simulink model "gm_sampleModel1569_sub"  (R2023a)
settings: Solver=VariableStepAuto  StartTime=0.0  StopTime=10.0  RelTol=1e-3
libraries: hdlsllib x2, simulink x1
settings Model: Creator=user1  LastModifiedBy=user1
settings OptimizationCC: BlockReduction=off  ConditionallyExecuteInputs=off
settings DebuggingCC: InheritedTsInSrcMsg=none

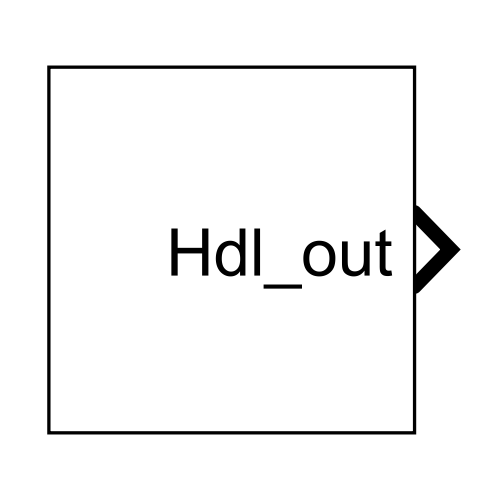
[thumbnail: Simulink's stored preview of the top-level diagram]
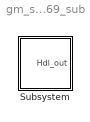
== system gm_sampleModel1569_sub ==
  Subsystem : Subsystem

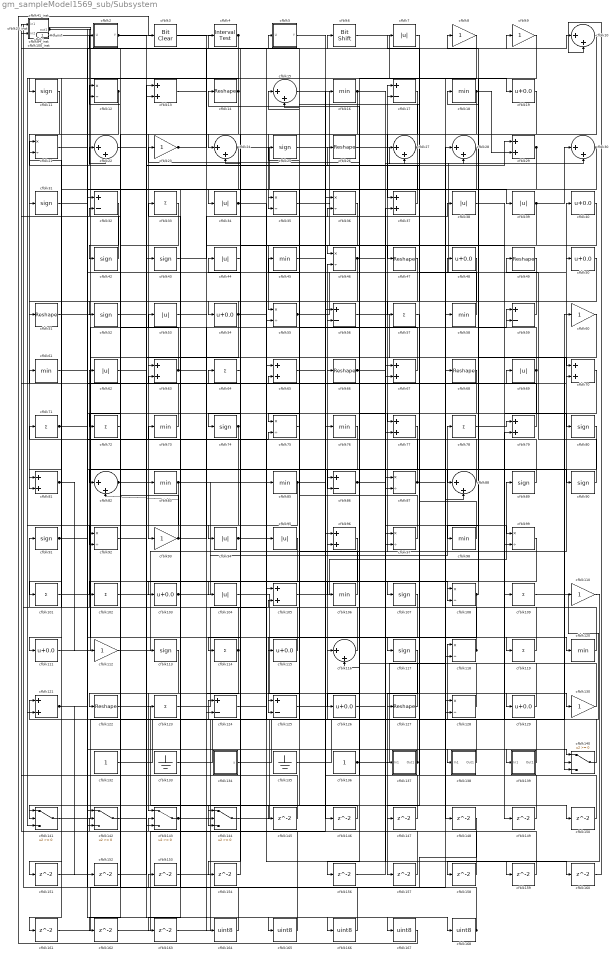
== system gm_sampleModel1569_sub/Subsystem ==
  cfblk1 : Constant  Value=0  OutDataTypeStr=uint8  SampleTime=1
  cfblk{10,15,22,24,27..28,30,82,88,116} (10 alike) : Sum  Inputs=|++  OutDataTypeStr=uint8
  cfblk100_inst : Subsystem
  cfblk{33,57,64,71..72,78,101..102,109,114,119,123} (12 alike) : Sum  Inputs=+  OutDataTypeStr=uint8
  cfblk{19,40,48,50,54,103,111,115,126,129} (10 alike) : Bias  Bias=0.0  SaturateOnIntegerOverflow=off
  cfblk{7,34,38..39,44,53,62,69,94..95,104} (11 alike) : Abs  OutDataTypeStr=uint8  SaturateOnIntegerOverflow=off
  cfblk{13,29,37,63,65,67,70,77,79,81,96,105,121} (13 alike) : Sum  OutDataTypeStr=uint8
  cfblk{16,18,45,58,61,73,76,83,85,98,106,120} (12 alike) : MinMax  OutDataTypeStr=uint8
  cfblk{11,25,31,42..43,52,74,80,89..91,107,113,117} (14 alike) : Signum
  cfblk{12,21,35..36,46,55,75,87,92,97,99,108,118,128} (14 alike) : Product  Inputs=*/  OutDataTypeStr=uint8  RndMeth=Zero  SaturateOnIntegerOverflow=on
  cfblk{8..9,23,60,93,110,112,130} (8 alike) : Gain  OutDataTypeStr=uint8
  cfblk{14,26,47,49,51,66,68,122,127} (9 alike) : Reshape
  cfblk{17,32,56,59,86,124..125} (7 alike) : Sum  Inputs=+-  OutDataTypeStr=uint8
  cfblk132 : Constant  OutDataTypeStr=uint8  SampleTime=-1
  cfblk133 : Ground
  cfblk134 : Subsystem  mask(Counter Free-Running){NumBits=double(16), tsamp=double(-1)}
      mask prompts: NumBits "Simulink:masks:NumberOfBits_MP"; tsamp "Simulink:masks:SampleTime_MP"
      mask help: Simulink:masks:CounterFreeRunning_MD
  cfblk135 : Ground
  cfblk136 : Constant  OutDataTypeStr=uint8  SampleTime=-1
  cfblk137 : Subsystem
  cfblk138 : Subsystem
  cfblk139 : Subsystem
  cfblk{140..144} (5 alike) : Switch  OutDataTypeStr=uint8  SaturateOnIntegerOverflow=off  InputSameDT=off
  cfblk{145..154,156..163} (18 alike) : Delay  SampleTime=1
  cfblk{164..168} (5 alike) : DataTypeConversion  OutDataTypeStr=uint8  SaturateOnIntegerOverflow=off  RndMeth=Floor
  cfblk2 : Subsystem  mask(Detect Fall Negative){vinit=double(0), InputProcessing=Elements as channels (sample based), OutDataTypeStr=uint8}
      mask prompts: vinit "Simulink:masks:InitialCondition_MP"; InputProcessing "Simulink:masks:InputProcessing_MP"; OutDataTypeStr "Simulink:masks:OutputDataType_MP"
      mask help: Simulink:masks:DetectFallNegative_MD
      mask init:
      | InputProcessing = 'Elements as channels (sample based)';
      | OutDataTypeStr = 'uint8';
      | vinit = double(0);
      mask TypeOptions InputProcessing: Simulink:masks:ColumnsAsChannelsFrameBased | Simulink:masks:ElementsAsChannelsSampleBased
      mask TypeOptions OutDataTypeStr: Simulink:masks:uint8 | Simulink:masks:boolean
      mask Display: fprintf('U < 0\n&  NOT\nU/z < 0')
  cfblk20_inst : Subsystem
  cfblk3 : simulink/Logic and Bit Operations/Bit Clear  iBit=0
      settings: LibrarySourceBlock=|
      | hdlsllib/Logic and Bit
      | Operations/Bit Clear
  cfblk4 : hdlsllib/Logic and Bit Operations/Interval Test  IntervalClosedRight=on  uplimit=0.5  IntervalClosedLeft=on  lowlimit=-0.5  OutDataTypeStr=uint8
  cfblk41_inst : Subsystem
  cfblk5 : Subsystem  mask(Detect Fall Negative){vinit=double(0), InputProcessing=Elements as channels (sample based), OutDataTypeStr=uint8}
      mask prompts: vinit "Simulink:masks:InitialCondition_MP"; InputProcessing "Simulink:masks:InputProcessing_MP"; OutDataTypeStr "Simulink:masks:OutputDataType_MP"
      mask help: Simulink:masks:DetectFallNegative_MD
      mask init:
      | InputProcessing = 'Elements as channels (sample based)';
      | OutDataTypeStr = 'uint8';
      | vinit = double(0);
      mask TypeOptions InputProcessing: Simulink:masks:ColumnsAsChannelsFrameBased | Simulink:masks:ElementsAsChannelsSampleBased
      mask TypeOptions OutDataTypeStr: Simulink:masks:uint8 | Simulink:masks:boolean
      mask Display: fprintf('U < 0\n&  NOT\nU/z < 0')
  cfblk6 : hdlsllib/Logic and Bit Operations/Bit Shift  mode=Shift Left Logical  N=0
  cfblk84_inst : Subsystem
  Hdl_out : Outport  OutDataTypeStr=uint8  SampleTime=1
  wires:
  cfblk1/1 -> cfblk19/1
  cfblk10/1 -> cfblk93/1
  cfblk100_inst/1(out1) -> cfblk22/2, cfblk120/1
  cfblk101/1 -> cfblk53/1
  cfblk102/1 -> cfblk17/1
  cfblk103/1 -> cfblk78/1, cfblk85/1
  cfblk104/1 -> cfblk129/1
  cfblk105/1 -> cfblk89/1
  cfblk106/1 -> cfblk65/2
  cfblk107/1 -> cfblk117/1
  cfblk108/1 -> cfblk125/2, cfblk8/1
  cfblk109/1 -> cfblk121/1
  cfblk11/1 -> cfblk81/2
  cfblk110/1 -> cfblk158/1
  cfblk111/1 -> cfblk64/1
  cfblk112/1 -> cfblk40/1
  cfblk113/1 -> cfblk122/1
  cfblk114/1 -> cfblk143/1, cfblk100_inst/1(in1)
  cfblk115/1 -> cfblk62/1
  cfblk116/1 -> cfblk71/1
  cfblk117/1 -> cfblk157/1
  cfblk118/1 -> cfblk91/1, cfblk44/1
  cfblk119/1 -> cfblk65/1
  cfblk12/1 -> cfblk31/1, cfblk101/1
  cfblk120/1 -> cfblk105/2
  cfblk121/1 -> cfblk75/2, cfblk152/1
  cfblk122/1 -> cfblk150/1
  cfblk123/1 -> cfblk105/1
  cfblk124/1 -> cfblk95/1
  cfblk125/1 -> cfblk46/2
  cfblk126/1 -> cfblk67/2
  cfblk127/1 -> cfblk14/1
  cfblk128/1 -> cfblk23/1
  cfblk129/1 -> cfblk61/1
  cfblk13/1 -> cfblk138/1(In1)
  cfblk130/1 -> cfblk96/2
  cfblk132/1 -> cfblk60/1
  cfblk133/1 -> cfblk67/1
  cfblk134/1(y) -> cfblk118/1
  cfblk135/1 -> cfblk99/2
  cfblk136/1 -> cfblk66/1, cfblk58/1
  cfblk137/1(Out1) -> cfblk32/2, cfblk4/1
  cfblk138/1(Out1) -> cfblk116/1
  cfblk139/1(Out1) -> cfblk15/2
  cfblk14/1 -> cfblk11/1, cfblk92/2
  cfblk140/1 -> cfblk22/1
  cfblk141/1 -> cfblk43/1
  cfblk142/1 -> cfblk124/1
  cfblk143/1 -> cfblk79/2, cfblk110/1
  cfblk144/1 -> cfblk87/1
  cfblk145/1 -> cfblk84_inst/1(in1)
  cfblk146/1 -> cfblk141/2
  cfblk147/1 -> cfblk116/2
  cfblk148/1 -> cfblk142/2
  cfblk149/1 -> cfblk96/1
  cfblk15/1 -> cfblk148/1
  cfblk150/1 -> cfblk17/2
  cfblk151/1 -> cfblk142/3
  cfblk152/1 -> cfblk13/2
  cfblk153/1 -> cfblk55/2
  cfblk154/1 -> cfblk24/2
  cfblk156/1 -> cfblk37/2
  cfblk157/1 -> cfblk12/1
  cfblk158/1 -> cfblk41_inst/1(in1)
  cfblk159/1 -> cfblk63/2
  cfblk16/1 -> cfblk39/1, cfblk30/2, cfblk92/1, cfblk35/2
  cfblk160/1 -> cfblk10/2
  cfblk161/1 -> cfblk128/1
  cfblk162/1 -> cfblk36/1
  cfblk163/1 -> cfblk28/1
  cfblk164/1 -> cfblk153/1
  cfblk165/1 -> cfblk20_inst/1(in1)
  cfblk166/1 -> cfblk20_inst/2(in2)
  cfblk167/1 -> cfblk3/1
  cfblk168/1 -> cfblk32/1, cfblk143/2
  cfblk17/1 -> cfblk37/1
  cfblk18/1 -> cfblk94/1, cfblk29/2, cfblk128/2
  cfblk19/1 -> cfblk24/1
  cfblk2/1(Y) -> cfblk165/1, cfblk108/2
  cfblk20_inst/1(out1) -> cfblk164/1
  cfblk21/1 -> cfblk35/1
  cfblk22/1 -> cfblk113/1
  cfblk23/1 -> cfblk47/1, cfblk10/1
  cfblk24/1 -> cfblk88/2, cfblk63/1
  cfblk25/1 -> cfblk97/1
  cfblk26/1 -> cfblk27/2
  cfblk27/1 -> cfblk74/1, cfblk41_inst/2(in2)
  cfblk28/1 -> cfblk34/1
  cfblk29/1 -> cfblk75/1, cfblk145/1
  cfblk3/1 -> cfblk168/1
  cfblk30/1 -> cfblk126/1, cfblk111/1
  cfblk31/1 -> cfblk90/1
  cfblk32/1 -> cfblk42/1
  cfblk33/1 -> cfblk72/1
  cfblk34/1 -> cfblk144/3, cfblk130/1
  cfblk35/1 -> cfblk149/1
  cfblk36/1 -> cfblk55/1
  cfblk37/1 -> cfblk13/1
  cfblk38/1 -> cfblk80/1
  cfblk39/1 -> cfblk30/1, cfblk114/1
  cfblk4/1 -> cfblk141/3, cfblk141/1, cfblk124/2, Hdl_out/1
  cfblk40/1 -> cfblk54/1
  cfblk41_inst/1(out1) -> cfblk83/1
  cfblk42/1 -> cfblk84_inst/2(in2)
  cfblk43/1 -> cfblk36/2
  cfblk44/1 -> cfblk144/1
  cfblk45/1 -> cfblk146/1
  cfblk46/1 -> cfblk70/1, cfblk123/1
  cfblk47/1 -> cfblk115/1
  cfblk48/1 -> cfblk81/1
  cfblk49/1 -> cfblk156/1
  cfblk5/1(Y) -> cfblk76/1
  cfblk50/1 -> cfblk118/2
  cfblk51/1 -> cfblk109/1
  cfblk52/1 -> cfblk26/1
  cfblk53/1 -> cfblk107/1
  cfblk54/1 -> cfblk6/1, cfblk56/2, cfblk51/1, cfblk143/3, cfblk160/1
  cfblk55/1 -> cfblk28/2, cfblk87/2
  cfblk56/1 -> cfblk140/2
  cfblk57/1 -> cfblk77/1
  cfblk58/1 -> cfblk27/1
  cfblk59/1 -> cfblk52/1
  cfblk6/1 -> cfblk68/1
  cfblk60/1 -> cfblk98/1
  cfblk61/1 -> cfblk167/1
  cfblk62/1 -> cfblk88/1
  cfblk63/1 -> cfblk127/1, cfblk2/1(U), cfblk137/1(In1)
  cfblk64/1 -> cfblk154/1
  cfblk65/1 -> cfblk16/1
  cfblk66/1 -> cfblk86/2, cfblk59/1
  cfblk67/1 -> cfblk5/1(U)
  cfblk68/1 -> cfblk86/1
  cfblk69/1 -> cfblk97/2, cfblk18/1
  cfblk7/1 -> cfblk57/1
  cfblk70/1 -> cfblk147/1
  cfblk71/1 -> cfblk69/1, cfblk139/1(In1)
  cfblk72/1 -> cfblk162/1
  cfblk73/1 -> cfblk12/2
  cfblk74/1 -> cfblk82/1, cfblk151/1
  cfblk75/1 -> cfblk45/1
  cfblk76/1 -> cfblk144/2
  cfblk77/1 -> cfblk163/1
  cfblk78/1 -> cfblk79/1
  cfblk79/1 -> cfblk100_inst/2(in2)
  cfblk8/1 -> cfblk46/1
  cfblk80/1 -> cfblk125/1
  cfblk81/1 -> cfblk161/1, cfblk112/1
  cfblk82/1 -> cfblk56/1, cfblk140/1
  cfblk83/1 -> cfblk50/1, cfblk121/2, cfblk33/1
  cfblk84_inst/1(out1) -> cfblk77/2, cfblk142/1, cfblk119/1
  cfblk85/1 -> cfblk38/1, cfblk104/1
  cfblk86/1 -> cfblk99/1, cfblk159/1
  cfblk87/1 -> cfblk140/3, cfblk21/1
  cfblk88/1 -> cfblk25/1
  cfblk89/1 -> cfblk73/1
  cfblk9/1 -> cfblk108/1
  cfblk90/1 -> cfblk49/1
  cfblk91/1 -> cfblk48/1, cfblk9/1
  cfblk92/1 -> cfblk166/1
  cfblk93/1 -> cfblk82/2, cfblk59/2, cfblk21/2
  cfblk94/1 -> cfblk70/2, cfblk29/1
  cfblk95/1 -> cfblk102/1
  cfblk96/1 -> cfblk103/1
  cfblk97/1 -> cfblk15/1
  cfblk98/1 -> cfblk7/1
  cfblk99/1 -> cfblk106/1

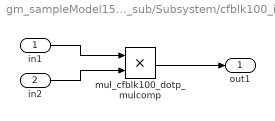
== system gm_sampleModel1569_sub/Subsystem/cfblk100_inst ==
  in1 : Inport  OutDataTypeStr=uint8  SampleTime=1
  in2 : Inport  Port=2  OutDataTypeStr=uint8  SampleTime=1
  mul_cfblk100_dotp_mulcomp : Product  Inputs=**  OutDataTypeStr=uint8  SampleTime=1
  out1 : Outport  OutDataTypeStr=uint8  SampleTime=1
  wires:
  in1/1 -> mul_cfblk100_dotp_mulcomp/1
  in2/1 -> mul_cfblk100_dotp_mulcomp/2
  mul_cfblk100_dotp_mulcomp/1 -> out1/1

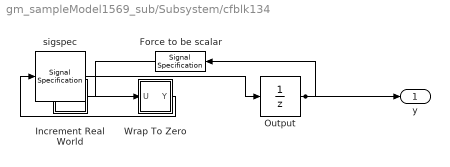
== system gm_sampleModel1569_sub/Subsystem/cfblk134 ==
  Force to be scalar : SignalSpecification  DisableCoverage=on  Dimensions=1
  Increment Real World : Subsystem  mask(Real World Value Increment){}
      mask help: Simulink:masks:RealWorldValueIncrement_MD
      mask Display: disp('V++')
  Output : UnitDelay  InitialCondition=0.0  SampleTime=tsamp  HasFrameUpgradeWarning=on
  Wrap To Zero : Subsystem  mask(Wrap To Zero){Threshold=double(65535)}
      mask prompts: Threshold "Simulink:masks:Threshold_MP"
      mask help: Simulink:masks:WrapToZero_MD
  sigspec : SignalSpecification  OutDataTypeStr=uint16  Dimensions=1
  y : Outport  SampleTime=1
  wires:
  Force to be scalar/1 -> Increment Real World/1(u)
  Increment Real World/1(y) -> Wrap To Zero/1(U)
  Output/1 -> Force to be scalar/1, y/1
  Wrap To Zero/1(Y) -> sigspec/1
  sigspec/1 -> Output/1

== system gm_sampleModel1569_sub/Subsystem/cfblk137 ==
  In1 : Inport  OutDataTypeStr=uint8  PortDimensions=1  SampleTime=1
  Out1 : Outport  SampleTime=1
  wires:
  In1/1 -> Out1/1

== system gm_sampleModel1569_sub/Subsystem/cfblk138 ==
  In1 : Inport  OutDataTypeStr=uint8  PortDimensions=1  SampleTime=1
  Out1 : Outport  SampleTime=1
  wires:
  In1/1 -> Out1/1

== system gm_sampleModel1569_sub/Subsystem/cfblk139 ==
  In1 : Inport  OutDataTypeStr=uint8  PortDimensions=1  SampleTime=1
  Out1 : Outport  SampleTime=1
  wires:
  In1/1 -> Out1/1

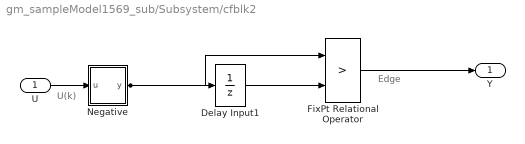
== system gm_sampleModel1569_sub/Subsystem/cfblk2 ==
  note: U(k)
  note: Edge
  U : Inport  OutDataTypeStr=uint8  SampleTime=1
  Delay Input1 : UnitDelay  Description=Store in Global RAM  DisableCoverage=on  InitialCondition=vinit  SampleTime=-1  HasFrameUpgradeWarning=on
  FixPt Relational Operator : RelationalOperator  Operator=>  OutDataTypeStr=fixdt(0, 8)  ZeroCross=off  InputSameDT=off
  Negative : Subsystem  mask(Compare To Zero){relop=<, OutDataTypeStr=boolean, ZeroCross=off}
      mask prompts: relop "Simulink:masks:Operator_MP"; OutDataTypeStr "Simulink:masks:OutputDataType_MP"; ZeroCross "Simulink:masks:EnableZerocrossingDetection_MP"
      mask help: Simulink:masks:CompareToZero_MD
      mask init:
      | OutDataTypeStr = 'boolean';
      | ZeroCross = 'off';
      | blkName = 'sampleModel1569_sub/Subsystem/cfblk2/Negative';
      | relop = '<';
      | setValue = 'boolean';
      mask TypeOptions relop: == | ~= | < | <= | >= | >
      mask TypeOptions OutDataTypeStr: Simulink:masks:uint8 | Simulink:masks:boolean
      mask Callback ZeroCross: sl('zeroCrossEnable', gcbh);
      mask Display: disp([relop,' 0'])
  Y : Outport  SampleTime=1
  wires:
  U/1 -> Negative/1(u)
  Delay Input1/1 -> FixPt Relational Operator/2
  FixPt Relational Operator/1 -> Y/1
  Negative/1(y) -> FixPt Relational Operator/1, Delay Input1/1

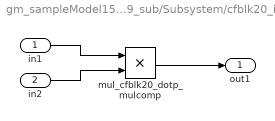
== system gm_sampleModel1569_sub/Subsystem/cfblk20_inst ==
  in1 : Inport  OutDataTypeStr=uint8  SampleTime=1
  in2 : Inport  Port=2  OutDataTypeStr=uint8  SampleTime=1
  mul_cfblk20_dotp_mulcomp : Product  Inputs=**  OutDataTypeStr=uint8  SampleTime=1
  out1 : Outport  OutDataTypeStr=uint8  SampleTime=1
  wires:
  in1/1 -> mul_cfblk20_dotp_mulcomp/1
  in2/1 -> mul_cfblk20_dotp_mulcomp/2
  mul_cfblk20_dotp_mulcomp/1 -> out1/1

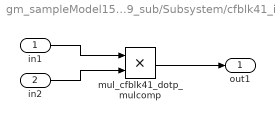
== system gm_sampleModel1569_sub/Subsystem/cfblk41_inst ==
  in1 : Inport  OutDataTypeStr=uint8  SampleTime=1
  in2 : Inport  Port=2  OutDataTypeStr=uint8  SampleTime=1
  mul_cfblk41_dotp_mulcomp : Product  Inputs=**  OutDataTypeStr=uint8  SampleTime=1
  out1 : Outport  OutDataTypeStr=uint8  SampleTime=1
  wires:
  in1/1 -> mul_cfblk41_dotp_mulcomp/1
  in2/1 -> mul_cfblk41_dotp_mulcomp/2
  mul_cfblk41_dotp_mulcomp/1 -> out1/1

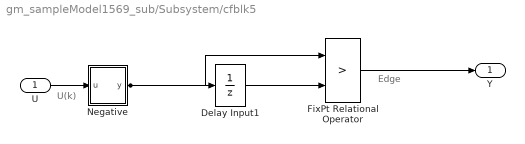
== system gm_sampleModel1569_sub/Subsystem/cfblk5 ==
  note: U(k)
  note: Edge
  U : Inport  OutDataTypeStr=uint8  SampleTime=1
  Delay Input1 : UnitDelay  Description=Store in Global RAM  DisableCoverage=on  InitialCondition=vinit  SampleTime=-1  HasFrameUpgradeWarning=on
  FixPt Relational Operator : RelationalOperator  Operator=>  OutDataTypeStr=fixdt(0, 8)  ZeroCross=off  InputSameDT=off
  Negative : Subsystem  mask(Compare To Zero){relop=<, OutDataTypeStr=boolean, ZeroCross=off}
      mask prompts: relop "Simulink:masks:Operator_MP"; OutDataTypeStr "Simulink:masks:OutputDataType_MP"; ZeroCross "Simulink:masks:EnableZerocrossingDetection_MP"
      mask help: Simulink:masks:CompareToZero_MD
      mask init:
      | OutDataTypeStr = 'boolean';
      | ZeroCross = 'off';
      | blkName = 'sampleModel1569_sub/Subsystem/cfblk5/Negative';
      | relop = '<';
      | setValue = 'boolean';
      mask TypeOptions relop: == | ~= | < | <= | >= | >
      mask TypeOptions OutDataTypeStr: Simulink:masks:uint8 | Simulink:masks:boolean
      mask Callback ZeroCross: sl('zeroCrossEnable', gcbh);
      mask Display: disp([relop,' 0'])
  Y : Outport  SampleTime=1
  wires:
  U/1 -> Negative/1(u)
  Delay Input1/1 -> FixPt Relational Operator/2
  FixPt Relational Operator/1 -> Y/1
  Negative/1(y) -> FixPt Relational Operator/1, Delay Input1/1

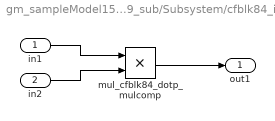
== system gm_sampleModel1569_sub/Subsystem/cfblk84_inst ==
  in1 : Inport  OutDataTypeStr=uint8  SampleTime=1
  in2 : Inport  Port=2  OutDataTypeStr=uint8  SampleTime=1
  mul_cfblk84_dotp_mulcomp : Product  Inputs=**  OutDataTypeStr=uint8  SampleTime=1
  out1 : Outport  OutDataTypeStr=uint8  SampleTime=1
  wires:
  in1/1 -> mul_cfblk84_dotp_mulcomp/1
  in2/1 -> mul_cfblk84_dotp_mulcomp/2
  mul_cfblk84_dotp_mulcomp/1 -> out1/1

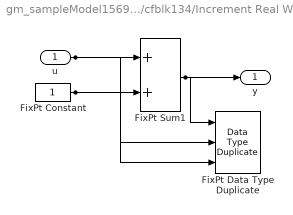
== system gm_sampleModel1569_sub/Subsystem/cfblk134/Increment Real World ==
  u : Inport  OutDataTypeStr=uint16  SampleTime=1
  FixPt Constant : Constant  DisableCoverage=on  OutDataTypeStr=Inherit: Inherit via back propagation  SampleTime=-1
  FixPt Data Type Duplicate : DataTypeDuplicate  DisableCoverage=on  NumInputPorts=3
  FixPt Sum1 : Sum  InputSameDT=on  OutDataTypeStr=Inherit: Inherit via back propagation  LockScale=on
  y : Outport  SampleTime=1
  wires:
  u/1 -> FixPt Sum1/1, FixPt Data Type Duplicate/2
  FixPt Constant/1 -> FixPt Sum1/2, FixPt Data Type Duplicate/3
  FixPt Sum1/1 -> FixPt Data Type Duplicate/1, y/1

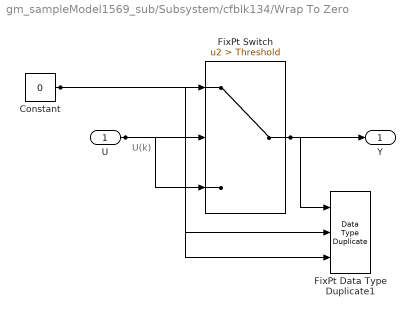
== system gm_sampleModel1569_sub/Subsystem/cfblk134/Wrap To Zero ==
  note: U(k)
  U : Inport  OutDataTypeStr=uint16  SampleTime=1
  Constant : Constant  DisableCoverage=on  Value=0  OutDataTypeStr=Inherit: Inherit via back propagation  SampleTime=-1
  FixPt Data Type Duplicate1 : DataTypeDuplicate  DisableCoverage=on  NumInputPorts=3
  FixPt Switch : Switch  Criteria=u2 > Threshold  Threshold=Threshold  OutDataTypeStr=Inherit: Inherit via back propagation  ZeroCross=off  SaturateOnIntegerOverflow=off  InputSameDT=off
  Y : Outport  SampleTime=1
  wires:
  U/1 -> FixPt Switch/3, FixPt Switch/2, FixPt Data Type Duplicate1/2
  Constant/1 -> FixPt Switch/1, FixPt Data Type Duplicate1/3
  FixPt Switch/1 -> FixPt Data Type Duplicate1/1, Y/1

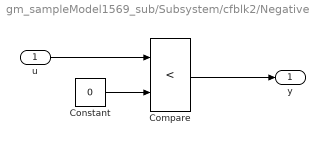
== system gm_sampleModel1569_sub/Subsystem/cfblk2/Negative ==
  u : Inport  OutDataTypeStr=uint8  SampleTime=1
  Compare : RelationalOperator  Operator=<  OutDataTypeStr=boolean  ZeroCross=off
  Constant : Constant  DisableCoverage=on  Value=0  OutDataTypeStr=Inherit: Inherit via back propagation  SampleTime=-1  PreserveConstantTs=on
  y : Outport  SampleTime=1
  wires:
  u/1 -> Compare/1
  Compare/1 -> y/1
  Constant/1 -> Compare/2

== system gm_sampleModel1569_sub/Subsystem/cfblk5/Negative ==
  u : Inport  OutDataTypeStr=uint8  SampleTime=1
  Compare : RelationalOperator  Operator=<  OutDataTypeStr=boolean  ZeroCross=off
  Constant : Constant  DisableCoverage=on  Value=0  OutDataTypeStr=Inherit: Inherit via back propagation  SampleTime=-1  PreserveConstantTs=on
  y : Outport  SampleTime=1
  wires:
  u/1 -> Compare/1
  Compare/1 -> y/1
  Constant/1 -> Compare/2
